simulink model "simulink_testcode"  (R2015a)
settings: Solver=FixedStepDiscrete  StartTime=0.0  StopTime=0.149  FixedStep=Te  RelTol=1e-3
values from neighbouring files (symbols this model uses):
  ka = 0.1    [script.m]
  Te = 1e-3    (= 0.001)    [script.m]
settings Model: TunableVars=Te,ka  TunableVarsStorageClass=Auto,Auto  TunableVarsTypeQualifier=,  Creator=gemsdev  LastModifiedBy=Damien
settings DataIOCC: LoadExternalInput=on  SignalLoggingSaveFormat=ModelDataLogs
settings OptimizationCC: InlineParams=on  OptimizeModelRefInitCode=on  LifeSpan=1
settings DebuggingCC: UnderspecifiedInitializationDetection=Classic  MergeDetectMultiDrivingBlocksExec=none  SolverPrmCheckMsg=warning
settings RTWCC: SystemTargetFile=ert.tlc  TemplateMakefile=RTW.MSVCBuild  Description=Create Visual C/C++ Solution File for Embedded Coder  TargetLang=C++
settings CodeAppCC: IgnoreCustomStorageClasses=off
settings ERTTargetCC: ParMdlRefBuildCompliant=on  CompOptLevelCompliant=on  ConcurrentExecutionCompliant=on  ERTFirstTimeCompliant=on  SupportContinuousTime=off  SupportVariableSizeSignals=off  ModelStepFunctionPrototypeControlCompliant=on  CPPClassGenCompliant=on  ERTCustomFileTemplate=example_file_process.tlc

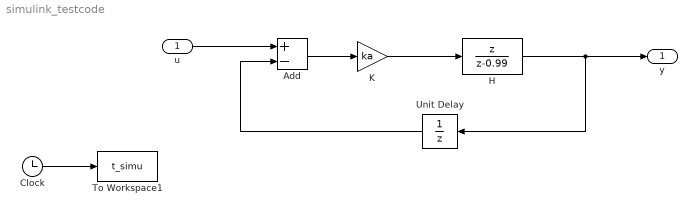
== system simulink_testcode ==
  u : Inport
  Add : Sum  Inputs=+-  SampleTime=Te
  Clock : Clock
  H : DiscreteTransferFcn  Numerator=[1 0]  Denominator=[1 -0.99]  SampleTime=Te
  K : Gain  Gain=ka  SampleTime=Te
  To Workspace1 : ToWorkspace  VariableName=t_simu  SampleTime=-1
  Unit Delay : UnitDelay  SampleTime=Te
  y : Outport
  wires:
  u/1 -> Add/1
  H/1 -> y/1, Unit Delay/1
  Unit Delay/1 -> Add/2
  Add/1 -> K/1
  K/1 -> H/1
  Clock/1 -> To Workspace1/1
